simulink model "LQ_PI_control_2015"  (R2020a)
settings: Solver=ode4  StartTime=0.0  StopTime=inf  FixedStep=0.002  RelTol=1e-3  EnableMultiTasking=on
undefined symbols (not defined in the file): gains_increasing, I_eq_increasing, K_pos_increasing_lq, K_vel_increasing_lq, Kp_i_increasing, Kp_lq_increasing, Ti_i_increasing, Ti_lq_increasing, x_eq, x_eq_increasing
libraries: PoliArd x6, simulink x6
settings Model: ExtModeTrigDuration=2  Creator=User  LastModifiedBy=miche
settings DataIOCC: LimitDataPoints=on  SaveFormat=Array  ReturnWorkspaceOutputs=off
settings OptimizationCC: LifeSpan=1  EfficientTunableParamExpr=on
settings DebuggingCC: UnderspecifiedInitializationDetection=Classic  MergeDetectMultiDrivingBlocksExec=none  SFUnexpectedBacktrackingDiag=warning  SFNoUnconditionalDefaultTransitionDiag=warning  SFExecutionAtInitializationDiag=none  ArithmeticOperatorsInVariantConditions=warning
settings HardwareCC: ProdBitPerPointer=32  ProdBitPerSizeT=32  ProdBitPerPtrDiffT=32  ProdLargestAtomicInteger=Long  ProdLargestAtomicFloat=Double  ProdIntDivRoundTo=Undefined  ProdWordSize=32  ProdHWDeviceType=ARM Compatible->ARM Cortex
settings ModelReferenceCC: PropagateSignalLabelsOutOfModel=off
settings SFSimCC: SimUseLocalCustomCode=off  MATLABDynamicMemAlloc=off  CustomCodeUndefinedFunction=UseInterfaceOnly
settings RTWCC: Description=Run on Target Hardware  SystemTargetFile=realtime.tlc  GenerateMakefile=off  TemplateMakefile=realtime.tmf  RTWVerbose=off  RTWUseLocalCustomCode=off
settings CodeAppCC: StateflowObjectComments=on
settings STFCustomTargetCC: TargetLibSuffix=.a  GenerateSampleERTMain=on  ERTCustomFileBanners=on  SupportNonInlinedSFcns=off  RemoveResetFunc=on  SupportVariableSizeSignals=on  MATLABClassNameForMDSCustomization=Simulink.SoftwareTarget.ERTCustomization  SystemTargetFile=realtime.tlc
settings ERTTargetCC: MultiwordLength=2048  GenerateSampleERTMain=on  ParMdlRefBuildCompliant=off  CompOptLevelCompliant=off  ConcurrentExecutionCompliant=off  CombineOutputUpdateFcns=off  SupportContinuousTime=on  SupportVariableSizeSignals=on  ModelStepFunctionPrototypeControlCompliant=off  CPPClassGenCompliant=off  UseToolchainInfoCompliant=off  ExtModeTransport=3  ExtModeMexFile=ext_serial_win32_comm_rtt  ExtModeMexArgs=0 1 9600  ERTSrcFileBannerTemplate=realtime_code_template.cgt  ERTHdrFileBannerTemplate=realtime_code_template.cgt  ERTDataSrcFileTemplate=realtime_code_template.cgt  ERTDataHdrFileTemplate=realtime_code_template.cgt  ERTCustomFileTemplate=realtime_file_process.tlc  ConvertIfToSwitch=off  SuppressUnreachableDefaultCases=off
settings ConfigComp: CovMetricSettings=dw  CovSaveCumulativeToWorkspaceVar=on  CovSaveSingleToWorkspaceVar=on  CovExternalEMLEnable=off

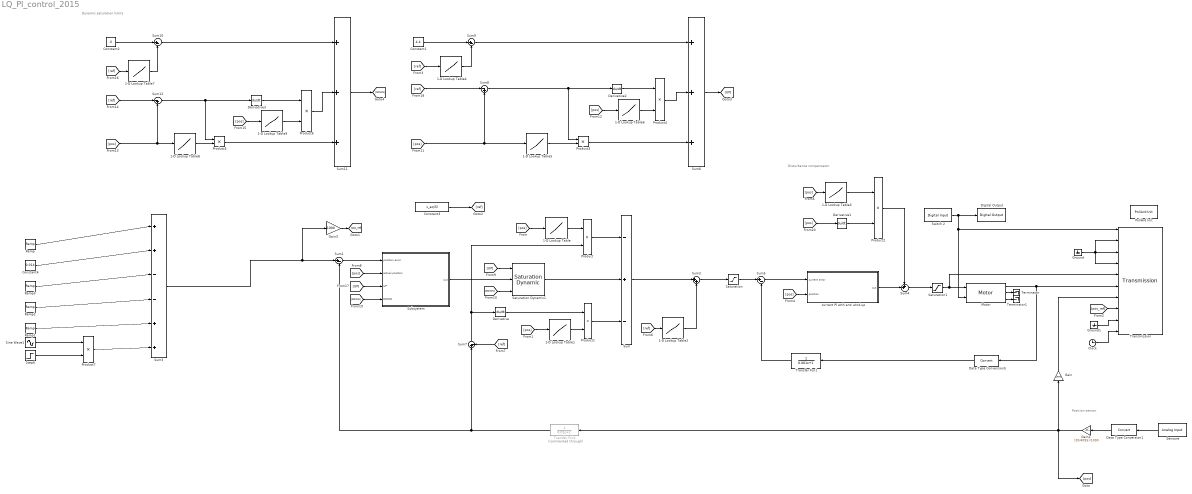
== system LQ_PI_control_2015 ==
  note: Disturbance compensator
  note: Position sensor
  note: Dynamic saturation limits
  1-D Lookup Table : Lookup_n-D  NumberOfTableDimensions=1  BreakpointsForDimension1=[0.0085 x_eq_increasing]  Table=[K_pos_increasing_lq(1) K_pos_increasing_lq]  InternalRulePriority=Speed  RndMeth=Simplest  InputSameDT=on
  1-D Lookup Table1 : Lookup_n-D  NumberOfTableDimensions=1  BreakpointsForDimension1=[0.0085 x_eq_increasing]  Table=[K_vel_increasing_lq(1) K_vel_increasing_lq]  InternalRulePriority=Speed  RndMeth=Simplest  InputSameDT=on
  1-D Lookup Table2 : Lookup_n-D  NumberOfTableDimensions=1  BreakpointsForDimension1=[0.0085 x_eq_increasing]  Table="[3.55  I_eq_increasing]"  InternalRulePriority=Speed  RndMeth=Simplest  InputSameDT=on
  1-D Lookup Table3 : Lookup_n-D  NumberOfTableDimensions=1  BreakpointsForDimension1=[0.0085 x_eq_increasing]  Table=[gains_increasing(1) gains_increasing]  InternalRulePriority=Speed  RndMeth=Simplest  InputSameDT=on
  1-D Lookup Table4 : Lookup_n-D  NumberOfTableDimensions=1  BreakpointsForDimension1=[0.0085 x_eq_increasing]  Table="[3.55  I_eq_increasing]"  InternalRulePriority=Speed  RndMeth=Simplest  InputSameDT=on
  1-D Lookup Table5 : Lookup_n-D  NumberOfTableDimensions=1  BreakpointsForDimension1=[0.0085 x_eq_increasing]  Table=[K_pos_increasing_lq(1) K_pos_increasing_lq]  InternalRulePriority=Speed  RndMeth=Simplest  InputSameDT=on
  1-D Lookup Table6 : Lookup_n-D  NumberOfTableDimensions=1  BreakpointsForDimension1=[0.0085 x_eq_increasing]  Table=[K_vel_increasing_lq(1) K_vel_increasing_lq]  InternalRulePriority=Speed  RndMeth=Simplest  InputSameDT=on
  1-D Lookup Table7 : Lookup_n-D  NumberOfTableDimensions=1  BreakpointsForDimension1=[0.0085 x_eq_increasing]  Table="[3.55  I_eq_increasing]"  InternalRulePriority=Speed  RndMeth=Simplest  InputSameDT=on
  1-D Lookup Table8 : Lookup_n-D  NumberOfTableDimensions=1  BreakpointsForDimension1=[0.0085 x_eq_increasing]  Table=[K_pos_increasing_lq(1) K_pos_increasing_lq]  InternalRulePriority=Speed  RndMeth=Simplest  InputSameDT=on
  1-D Lookup Table9 : Lookup_n-D  NumberOfTableDimensions=1  BreakpointsForDimension1=[0.0085 x_eq_increasing]  Table=[K_vel_increasing_lq(1) K_vel_increasing_lq]  InternalRulePriority=Speed  RndMeth=Simplest  InputSameDT=on
  Clock : Clock
  Constant1 : Constant  Value=4.4
  Constant2 : Constant  Value=0
  Constant3 : Constant  Value=x_eq(5)
  Constant4 : Constant  Value=0.014
  Data Type Conversion1 : DataTypeConversion
  Data Type Conversion5 : DataTypeConversion
  Derivative{,1..3} (4 alike) : Derivative
  Digital Output : PoliArd/Digital Output  DO_pin=1
  Gain : Gain  Gain=1000
  Gain1 : Gain  Gain=(20/4095)/1000
  Gain3 : Gain  Gain=1000
  Ground : Ground
  Ground1 : Ground
  Motor : PoliArd/Motor  MotorID=2  DC_bus_mask=24  dt_mot=-1
  PoliArd Init : PoliArd/PoliArd Init
  Product{,1..7} (8 alike) : Product
  Ramp : simulink/Sources/Ramp  slope=0.001  start=7  InitialOutput=0
  Ramp1 : simulink/Sources/Ramp  slope=0.001  start=18  InitialOutput=0
  Ramp2 : simulink/Sources/Ramp  slope=0.001  start=17  InitialOutput=0
  Ramp3 : simulink/Sources/Ramp  slope=0.001  start=10  InitialOutput=0
  Saturation : Saturate  UpperLimit=4.4  LowerLimit=0
  Saturation Dynamic1 : simulink/Discontinuities/Saturation Dynamic  OutMin=[]  OutMax=[]  OutDataTypeStr=Inherit: Same as second input  OutDataType=fixdt(1, 16)  OutScaling=2^-10  DoSatur=off
  Saturation1 : Saturate  UpperLimit=18  LowerLimit=0
  Sensore : PoliArd/Analog Input  AIpin_mask=2  AIsample=-1
  Sine Wave1 : Sin  Amplitude=0.002  Phase=0.3  SampleTime=0
  Step6 : Step  Time=28  SampleTime=0
  Subsystem : Subsystem
      mask Display: disp('Position controller\n(PI)\nwith anti wind-up')
  Sum : Sum  Inputs=-+-
  Sum{1,5,7,9..10} (5 alike) : Sum  Inputs=|+-
  Sum11 : Sum  Inputs=+++
  Sum12 : Sum  Inputs=|-+
  Sum2 : Sum  Inputs=|++
  Sum3 : Sum  Inputs=|++--++
  Sum4 : Sum  Inputs=++|
  Sum6 : Sum  Inputs=+++
  Sum8 : Sum  Inputs=|-+
  Switch 2 : PoliArd/Digital Input  DI_pin=2  DIsample=-1
  Terminator : Terminator
  Terminator1 : Terminator
  Transfer Fcn1 : TransferFcn  Denominator=[0.001 1]
  Transfer Fcn2 : TransferFcn  Commented=through  Denominator=[0.01 1]
  Transmission : PoliArd/Transmission  sample_freq=500  sig_to_send=6
  current PI with anti wind-up : Subsystem
      mask Display: disp('Current controller\n(PI)\nwith anti wind-up')
  wires:
  Switch 2/1 -> Motor/2, Transmission/1, Digital Output/1
  Sensore/1 -> Data Type Conversion1/1
  Ground/1 -> Transmission/4, Transmission/2, Transmission/3
  Motor/1 -> Transmission/6, Data Type Conversion5/1
  Data Type Conversion1/1 -> Gain1/1
  Gain1/1 -> Gain/1, [pos], Transfer Fcn2/1
  Gain/1 -> Transmission/7
  1-D Lookup Table4/1 -> Sum9/2
  1-D Lookup Table1/1 -> Product1/2
  Constant3/1 -> [ref]
  [DOWN] -> Saturation Dynamic1/3
  1-D Lookup Table/1 -> Product/1
  1-D Lookup Table7/1 -> Sum10/2
  Saturation/1 -> Sum5/1
  [pos] -> 1-D Lookup Table6/1
  Sum6/1 -> [UP]
  1-D Lookup Table8/1 -> Product5/2
  Derivative/1 -> Product1/1
  Product4/1 -> Sum6/2
  Transfer Fcn1/1 -> Sum5/2
  Sum11/1 -> [DOWN]
  [ref] -> 1-D Lookup Table7/1
  Derivative2/1 -> Product4/1
  Transfer Fcn2/1 -> Sum7/1, Sum1/2
  Product2/1 -> Sum4/1
  Saturation Dynamic1/1 -> Sum/2
  1-D Lookup Table3/1 -> Product2/1
  Product5/1 -> Sum11/3
  Constant1/1 -> Sum9/1
  [pos] -> 1-D Lookup Table3/1
  current PI with anti wind-up/1(out) -> Sum4/2
  Sum9/1 -> Sum6/1
  Product3/1 -> Sum6/3
  Subsystem/1(out) -> Saturation Dynamic1/2
  [pos] -> 1-D Lookup Table5/1, Sum8/2
  Sum4/1 -> Saturation1/1
  Product6/1 -> Sum11/2
  [ref] -> Sum7/2
  [ref] -> Sum12/1
  1-D Lookup Table6/1 -> Product4/2
  [pos] -> 1-D Lookup Table9/1
  1-D Lookup Table5/1 -> Product3/2
  Sum10/1 -> Sum11/1
  Sum7/1 -> Product/2, Derivative/1
  Sum/1 -> Sum2/1
  1-D Lookup Table9/1 -> Product6/2
  [pos] -> Sum12/2, 1-D Lookup Table8/1
  Sum12/1 -> Derivative3/1, Product5/1
  Sum1/1 -> Subsystem/1(position error)
  [ref] -> Sum8/1
  [pos] -> current PI with anti wind-up/2(position)
  [pos] -> 1-D Lookup Table1/1
  [UP] -> Saturation Dynamic1/1
  Derivative1/1 -> Product2/2
  Derivative3/1 -> Product6/1
  Product1/1 -> Sum/3
  Sum5/1 -> current PI with anti wind-up/1(current error)
  Product/1 -> Sum/1
  Sum2/1 -> Saturation/1
  [pos] -> Subsystem/2(actual position)
  [ref] -> 1-D Lookup Table2/1
  [pos] -> 1-D Lookup Table/1
  1-D Lookup Table2/1 -> Sum2/2
  Constant2/1 -> Sum10/1
  [ref] -> 1-D Lookup Table4/1
  Sum8/1 -> Product3/1, Derivative2/1
  [UP] -> Subsystem/3(UP)
  [DOWN] -> Subsystem/4(DOWN)
  Data Type Conversion5/1 -> Transfer Fcn1/1
  [pos] -> Derivative1/1
  Saturation1/1 -> Transmission/5, Motor/1
  Motor/2 -> Terminator/1
  Motor/3 -> Terminator1/1
  Gain3/1 -> [pos_ref]
  [pos_ref] -> Transmission/8
  Ground1/1 -> Transmission/9
  Clock/1 -> Transmission/10
  Ramp/1 -> Sum3/1
  Constant4/1 -> Sum3/2
  Ramp3/1 -> Sum3/3
  Ramp2/1 -> Sum3/4
  Ramp1/1 -> Sum3/5
  Sine Wave1/1 -> Product7/1
  Step6/1 -> Product7/2
  Product7/1 -> Sum3/6
  Sum3/1 -> Gain3/1, Sum1/1

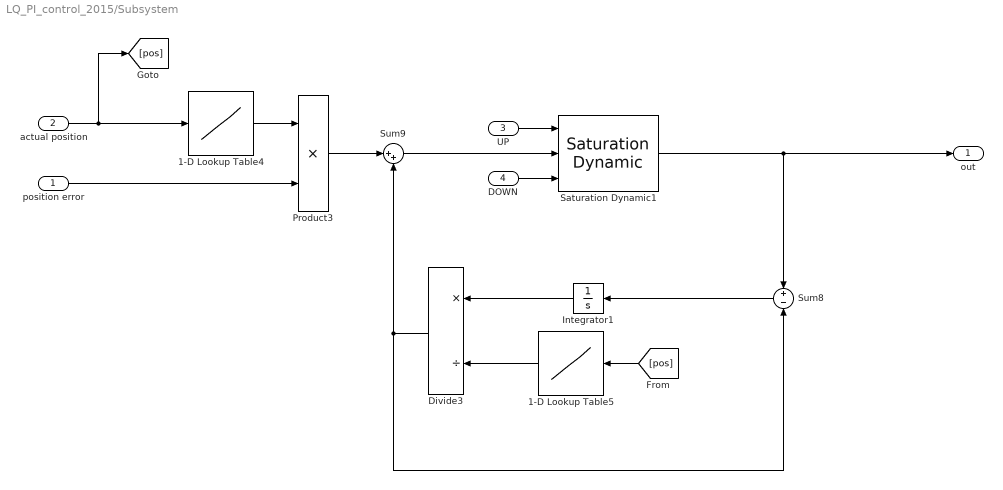
== system LQ_PI_control_2015/Subsystem ==
  position error : Inport
  actual position : Inport  Port=2
  UP : Inport  Port=3
  DOWN : Inport  Port=4
  1-D Lookup Table4 : Lookup_n-D  NumberOfTableDimensions=1  BreakpointsForDimension1=[0.0085 x_eq_increasing]  Table=[Kp_lq_increasing(1) Kp_lq_increasing]  InternalRulePriority=Speed  RndMeth=Simplest  InputSameDT=on
  1-D Lookup Table5 : Lookup_n-D  NumberOfTableDimensions=1  BreakpointsForDimension1=[0.0085 x_eq_increasing]  Table=[Ti_lq_increasing(1) Ti_lq_increasing]  InternalRulePriority=Speed  RndMeth=Simplest  InputSameDT=on
  Divide3 : Product  Inputs=*/
  Integrator1 : Integrator
  Product3 : Product
  Saturation Dynamic1 : simulink/Discontinuities/Saturation Dynamic  OutMin=[]  OutMax=[]  OutDataTypeStr=Inherit: Same as second input  OutDataType=fixdt(1, 16)  OutScaling=2^-10  DoSatur=off
  Sum8 : Sum  Inputs=+|-
  Sum9 : Sum  Inputs=|++
  out : Outport
  wires:
  Integrator1/1 -> Divide3/1
  Saturation Dynamic1/1 -> out/1, Sum8/1
  Product3/1 -> Sum9/1
  Sum9/1 -> Saturation Dynamic1/2
  1-D Lookup Table4/1 -> Product3/1
  Divide3/1 -> Sum8/2, Sum9/2
  Sum8/1 -> Integrator1/1
  position error/1 -> Product3/2
  1-D Lookup Table5/1 -> Divide3/2
  actual position/1 -> [pos], 1-D Lookup Table4/1
  [pos] -> 1-D Lookup Table5/1
  UP/1 -> Saturation Dynamic1/1
  DOWN/1 -> Saturation Dynamic1/3

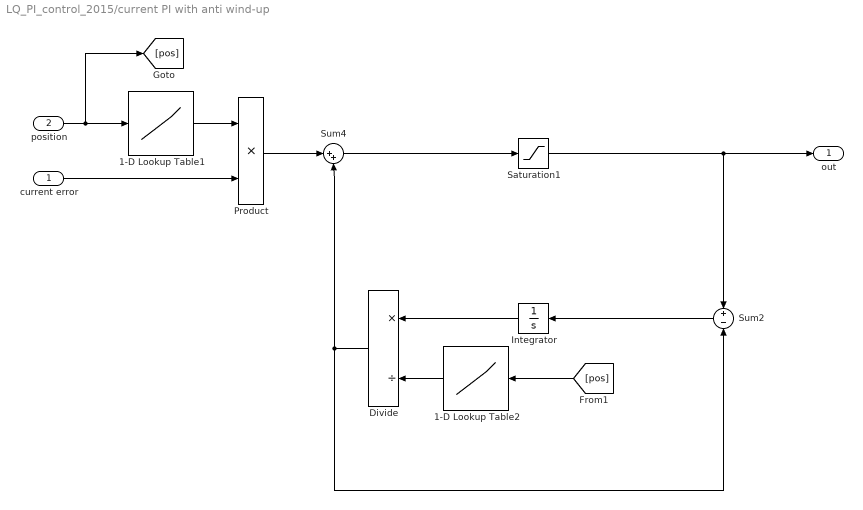
== system LQ_PI_control_2015/current PI with anti wind-up ==
  current error : Inport
  position : Inport  Port=2
  1-D Lookup Table1 : Lookup_n-D  NumberOfTableDimensions=1  BreakpointsForDimension1=[0.0085 x_eq_increasing]  Table=[Kp_i_increasing(1) Kp_i_increasing]  InternalRulePriority=Speed  RndMeth=Simplest  InputSameDT=on
  1-D Lookup Table2 : Lookup_n-D  NumberOfTableDimensions=1  BreakpointsForDimension1=[0.0085 x_eq_increasing]  Table=[Ti_i_increasing(1) Ti_i_increasing]  InternalRulePriority=Speed  RndMeth=Simplest  InputSameDT=on
  Divide : Product  Inputs=*/
  Integrator : Integrator
  Product : Product
  Saturation1 : Saturate  UpperLimit=18  LowerLimit=0
  Sum2 : Sum  Inputs=+|-
  Sum4 : Sum  Inputs=|++
  out : Outport
  wires:
  Sum4/1 -> Saturation1/1
  Product/1 -> Sum4/1
  Saturation1/1 -> out/1, Sum2/1
  1-D Lookup Table1/1 -> Product/1
  position/1 -> [pos], 1-D Lookup Table1/1
  Sum2/1 -> Integrator/1
  Integrator/1 -> Divide/1
  1-D Lookup Table2/1 -> Divide/2
  Divide/1 -> Sum2/2, Sum4/2
  current error/1 -> Product/2
  [pos] -> 1-D Lookup Table2/1
